simulink library "mbed_lib"  (Simulink 8.3)
settings: Solver=ode45  SolverMode=SingleTasking  StartTime=0.0  StopTime=10.0  RelTol=1e-3
settings Model: Creator=syoon  LastModifiedBy=oh

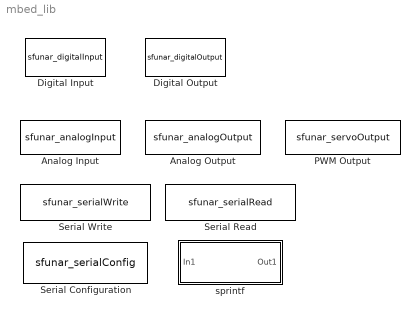
== system mbed_lib ==
  Analog Input : S-Function  FunctionName=sfunar_analogInput  Parameters=uint8(SParameter1), SampleTime, uint8(SParameter2)  EnableBusSupport=off  mask(Arduino Analog Input){SParameter2=A, SParameter1=0, SampleTime=-1}
      mask prompts: SParameter2 "Port Name:"; SParameter1 "Pin Number (1-16):"; SampleTime "Sample time (-1 for inherited):"
      mask help:
      | Reads the analog voltage input from the specified pin on the Arduino board.
      |
      | The range of input on the pin is between 0 and 5 Volts corresponding to a block output of 0 to 1023.
      mask Help:
      | <p>This block calls the analogRead() function from the Arduino language library.
      | <p>For more information see: <a href="http://arduino.cc/en/Reference/AnalogRead">Arduino - AnalogRead</a>
      mask TypeOptions SParameter2: A | B | C | D | E | F
      mask Display:
      | plot([0:0.05:0.5],0.3*sin(4*pi*[0.5:0.05:1])+0.5)
      | port_label('output',1,['Pin ', SParameter2+64, '.', num2str(SParameter1)]);
  Analog Output : S-Function  FunctionName=sfunar_analogOutput  Parameters=uint8(SParameter1), SampleTime, uint8(SParameter2)  EnableBusSupport=off  mask(Arduino Analog Output){SParameter2=A, SampleTime=-1, SParameter1=0}
      mask prompts: SParameter2 "Port Name:"; SampleTime "Sample time (-1 for inherited):"; SParameter1 "Pin Number (1-16):"
      mask help:
      | Approximates an analog output on the specified pin on the Arduino board using a PWM signal with a frequency of ~490 Hz.
      |
      | The input to this block is an integer between 0 and 255 corresponding to 0 to 5V.
      mask Help:
      | <p>This block calls the analogWrite() function from the Arduino language library.
      | <p>For more information see: <a href="http://arduino.cc/en/Reference/AnalogWrite">Arduino - AnalogWrite</a>
      mask TypeOptions SParameter2: A | B | C | D | E | F
      mask Display:
      | plot([0.5:0.05:1],0.3*sin(4*pi*[0.5:0.05:1])+0.5)
      | port_label('input',1,['Pin ', SParameter2+64, '.', num2str(SParameter1)]);
  Digital Input : S-Function  FunctionName=sfunar_digitalInput  Parameters=uint8(SParameter1), SampleTime, uint8(SParameter2), uint8(SParameter3)  EnableBusSupport=off  mask(Arduino Digital Input){SParameter2=A, SParameter1=0, SParameter3=INPUT, SampleTime=-1}
      mask prompts: SParameter2 "Port Name"; SParameter1 "Pin Number (1-16):"; SParameter3 "Input Mode"; SampleTime "Sample time (-1 for inherited):"
      mask help:
      | Reads the digital value from the specified pin on the Arduino board.
      |
      | It outputs 1 for high and 0 for low.
      mask Help:
      | <p>This block calls the digitalRead() function from the Arduino language library.
      | <p>For more information see: <a href="http://arduino.cc/en/Reference/DigitalRead">Arduino - DigitalRead</a>
      mask TypeOptions SParameter2: A | B | C | D | E | F
      mask TypeOptions SParameter3: INPUT | INPUT_PULLUP | INPUT_PULLDOWN
      mask Display:
      | plot([0 0.15 0.15 0.35 0.35 0.5],[0.3 0.3 0.7 0.7 0.3 0.3])
      | port_label('output',1,['Pin ', SParameter2+64, '.', num2str(SParameter1)]);
  Digital Output : S-Function  FunctionName=sfunar_digitalOutput  Parameters=uint8(SParameter1), SampleTime, uint8(SParameter2), uint8(SParameter3)  EnableBusSupport=off  mask(Arduino Digital Output){SParameter2=D, SParameter1=12, SParameter3=OUTPUT, SampleTime=-1}
      mask prompts: SParameter2 "Port Name:"; SParameter1 "Pin Number(1~16):"; SParameter3 "Output Mode"; SampleTime "Sample time (-1 for inherited):"
      mask help:
      | Sends the digital value to the specified port.pin on the Arduino board.
      | The pin can be configured as push-pull (pp) or open drain output (od).
      |
      | An input of 1 sets the pin high and 0 sets the pin low.
      mask Help:
      | <p>This block calls the digitalWrite() function from the Arduino language library.
      | <p>For init the pinmode function ist called
      | <p>For more information see: <a href="http://arduino.cc/en/Reference/DigitalWrite">Arduino - DigitalWrite</a>
      mask TypeOptions SParameter2: A | B | C | D | E | F
      mask TypeOptions SParameter3: OUTPUT | OUTPUT_OPENDRAIN
      mask Display:
      | plot([0.5 0.65 0.65 0.85 0.85 1],[0.3 0.3 0.7 0.7 0.3 0.3])
      | port_label('input',1,['Pin ', SParameter2+64, '.', num2str(SParameter1)]);
  PWM Output : S-Function  FunctionName=sfunar_servoOutput  Parameters=uint8(SParameter1), SampleTime  EnableBusSupport=off  mask(Arduino Analog Output){SParameter1=PA07 (TIM14_CH1), SampleTime=-1}
      mask prompts: SParameter1 "PWM Pin:"; SampleTime "Sample time (-1 for inherited):"
      mask help:
      | Approximates an analog output on the specified pin on the Arduino board using a PWM signal with a frequency of ~490 Hz.
      |
      | The input to this block is an integer between 0 and 255 corresponding to 0 to 5V.
      mask Help:
      | <p>This block calls the analogWrite() function from the Arduino language library.
      | <p>For more information see: <a href="http://arduino.cc/en/Reference/AnalogWrite">Arduino - AnalogWrite</a>
      mask TypeOptions SParameter1: PA07 (TIM14_CH1) | PA08 (TIM1_CH1) | PB00 (TIM3_CH3) | PB01 (TIM3_CH4) | PB04 (TIM3_CH1) | PB05 (TIM3_CH2) | PC06 (TIM8_CH1) | PC07 (TIM8_CH2) | PC08 (TIM8_CH3) | PC09 (TIM8_CH4) | PD12 (TIM4_CH1) | PD13 (TIM4_CH2) | PD14 (TIM4_CH3) | PD15 (TIM4_CH4) | PE13 (TIM1_CH3) | PE14 (TIM1_CH4)
      mask Display:
      | plot([0.5 0.65 0.65 0.85 ],[0.3 0.3 0.7 0.7 ])
      | plot([0.8 0.8],[0.7 0.3])
      | plot([0.825 0.825],[0.7 0.3])
      | plot([0.85 0.85],[0.7 0.3])
      | plot([0.8 1],[0.3 0.3])
      | p={'PA07';'PA08';'PB00';'PB01';'PB04';'PB05';'PC06';'PC07';'PC08';'PC09';'PD12';'PD13';'PD14';'PD15';'PE13';'PE14'};
      | port_label('input',1,[p{SParameter1}]);
  Serial Configuration : S-Function  FunctionName=sfunar_serialConfig  Parameters=uint8(SParameter1), uint8(SParameter2), uint8(SParameter3), uint8(SParameter4), uint8(SParameter5), SParameter6  EnableBusSupport=off  mask(Arduino Serial Configuration){SParameter1=1, SParameter6=9600, SParameter2=A, SParameter3=3, SParameter4=A, SParameter5=4}
      mask prompts: SParameter1 "Serial Port"; SParameter6 "Baud Rate:"; SParameter2 "Port Name (TX)"; SParameter3 "Pin Number (1-16):"; SParameter4 "Port Name (RX)"; SParameter5 "Pin Number (1-16):"
      mask help:
      | This blocks sets up the serial connection on the Arduino board. You must have one of these blocks in any model that ues the Serial Send or Serial Read blocks.
      |
      | Set the baud rate to match the device that you are communicating with. Standard rates include:300, 1200, 2400, 4800, 9600, 14400, 19200, 28800, 38400, 57600, or 115200.
      mask Help:
      | <p>This block calls the Serial.begin() function from the Arduino language library.
      | <p>For more information see: <a href="http://arduino.cc/en/Serial/Begin">Arduino - Serial/Begin</a>
      mask TypeOptions SParameter1: 1 | 2 | 3 | 4 | 5
      mask TypeOptions SParameter2: A | B | C | D | E | F
      mask TypeOptions SParameter3: 0 | 1 | 2 | 3 | 4 | 5 | 6 | 7 | 8 | 9 | 10 | 11 | 12 | 13 | 14 | 15
      mask TypeOptions SParameter4: A | B | C | D | E | F
      mask TypeOptions SParameter5: 0 | 1 | 2 | 3 | 4 | 5 | 6 | 7 | 8 | 9 | 10 | 11 | 12 | 13 | 14 | 15
      mask Display:
      | disp(['Serial Config ' num2str(SParameter1) '\n\n']);
      | disp(['TX ' SParameter2+64 '.' num2str(SParameter3-1) ', RX ' SParameter4+64, '.' num2str(SParameter5-1)]);
  Serial Read : S-Function  FunctionName=sfunar_serialRead  Parameters=SampleTime, uint8(SParameter1)  EnableBusSupport=off  mask(Arduino Serial Read){SParameter1=USB, SampleTime=-1}
      mask prompts: SParameter1 "Serial Port"; SampleTime "Sample time (-1 for inherited):"
      mask help:
      | Reads one byte from the serial interface on the Arduino board.
      |
      | Outputs -1 if no data is available to be read.
      mask Help:
      | <p>This block calls the Serial.read() function from the Arduino language library.
      | <p>For more information see: <a href="http://arduino.cc/en/Serial/Read">Arduino - Serial/Read</a>
      mask TypeOptions SParameter1: USB | UART1(A2,A3) | USART3(D8,D9)
      mask Display:
      | p={'USB'; 'UART1'; 'USART3'};
      | disp(['Serial Read ' p{SParameter1}])
  Serial Write : S-Function  FunctionName=sfunar_serialWrite  Parameters=SampleTime, uint8(SParameter1)  EnableBusSupport=off  mask(Arduino Serial Write){SParameter1=USB, SampleTime=-1}
      mask prompts: SParameter1 "Serial Port"; SampleTime "Sample time (-1 for inherited):"
      mask help:
      | Writes a vector of bytes to the serial port on the Arduino board.
      |
      | Outputs -1 if no data is available to be read.
      mask Help:
      | <p>This block calls the Serial.write() function from the Arduino language library.
      | <p>For more information see: <a href="http://arduino.cc/en/Serial/Write">Arduino - Serial/Write</a>
      mask TypeOptions SParameter1: USB | UART1(A2,A3) | USART3(D8,D9)
      mask Display:
      | p={'USB'; 'UART1'; 'USART3'};
      | disp(['Serial Write ' p{SParameter1}])
  sprintf : Subsystem  mask{format=%f}
      mask TypeOptions format: %f | %d
      mask Display:
      | p={'%f'; '%d'};
      | disp(['sprintf: ' p{format}])

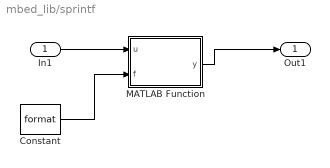
== system mbed_lib/sprintf ==
  In1 : Inport
  Constant : Constant  Value=format
  MATLAB Function : MATLAB Function  TreatAsAtomicUnit=on
  Out1 : Outport
  wires:
  In1/1 -> MATLAB Function/1(u)
  MATLAB Function/1(y) -> Out1/1
  Constant/1 -> MATLAB Function/2(f)

== matlab function sprintf/MATLAB Function ==
  data: u input double; y output double; f input double
function y = fcn(u,f)
buffer = char(zeros(1,15));
% geht mit 2012b noch nicht aber mit 2014a oder 2013: coder.cinclude('stdio.h');
coder.ceval('#ifdef _WIN32 //');
  if f == 1
    coder.ceval('_snprintf', coder.ref(buffer(int32(1))),int32(size(buffer,2)), ['%f' char(13) char(10) 0], u);
  elseif f==2
    coder.ceval('_snprintf', coder.ref(buffer(int32(1))),int32(size(buffer,2)), ['%d' char(13) char(10) 0], u);
  end
coder.ceval('#else //');
  if f == 1
    coder.ceval('snprintf', coder.ref(buffer(int32(1))),int32(size(buffer,2)), ['%f' char(13) char(10) 0], u);
  elseif f==2
    coder.ceval('snprintf', coder.ref(buffer(int32(1))),int32(size(buffer,2)), ['%d' char(13) char(10) 0], u);
  end
coder.ceval('#endif //');
y = uint8(buffer);
